simulink model "discrete_1ph_CL_VI"  (R2024a)
settings: Solver=VariableStepAuto  StartTime=0.0  StopTime=10.0  RelTol=1e-3
undefined symbols (not defined in the file): DiscIntNeverNeededParam, ILmax, kaw_i, kaw_v, ki_i, ki_v, kp_i, kp_v, Tsw, VinNom, VLlim, zden_aaf, zden_plant_i, znum_aaf, znum_plant_i
libraries: simulink x1
settings Model: Creator=marzu  LastModifiedBy=marzu

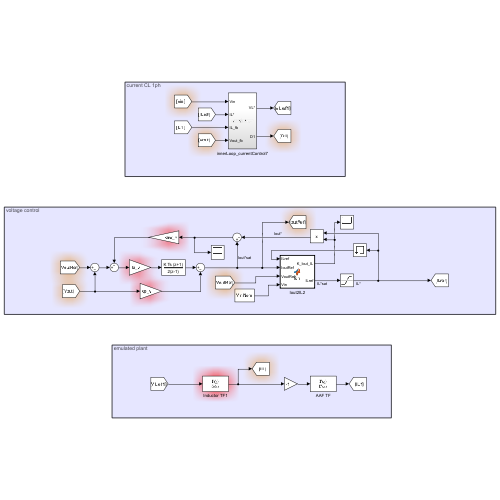
[thumbnail: Simulink's stored preview of the top-level diagram]
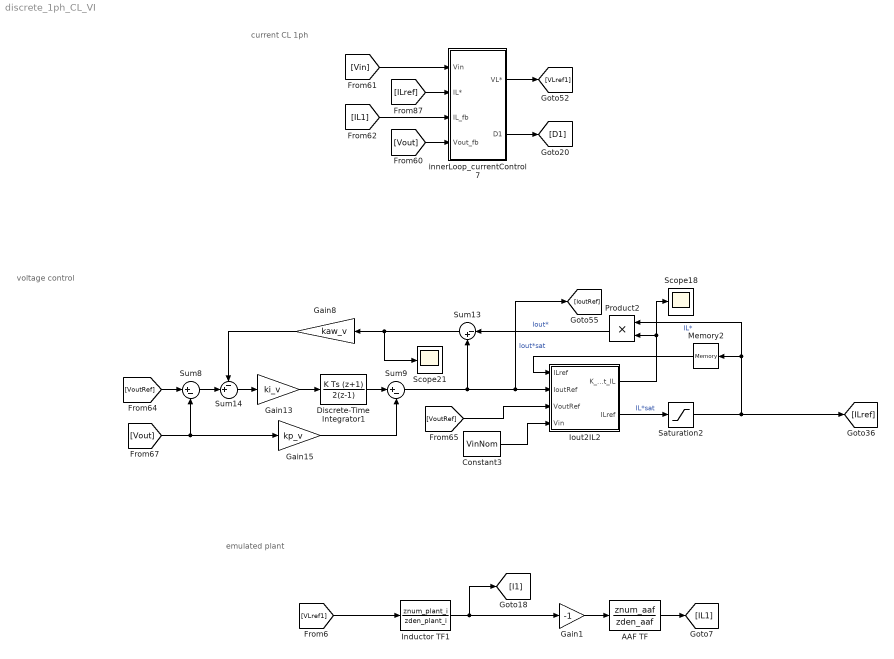
== system discrete_1ph_CL_VI ==
  note: voltage control
  note: emulated plant
  note: current CL 1ph
  AAF TF : DiscreteTransferFcn  Numerator=znum_aaf  Denominator=zden_aaf
  Constant3 : Constant  Value=VinNom
  Discrete-Time Integrator1 : DiscreteIntegrator  IntegratorMethod=Integration: Trapezoidal  SampleTime=Tsw  ICPrevOutput=DiscIntNeverNeededParam  ICPrevScaledInput=DiscIntNeverNeededParam
  Gain1 : Gain  Gain=-1
  Gain13 : Gain  Gain=ki_v
  Gain15 : Gain  Gain=kp_v
  Gain8 : Gain  Gain=kaw_v
  Inductor TF1 : DiscreteTransferFcn  Numerator=znum_plant_i  Denominator=zden_plant_i
  Iout2IL2 : MATLAB Function  TreatAsAtomicUnit=on
  Memory2 : Memory
  Product2 : Product
  Saturation2 : Saturate  UpperLimit=ILmax  LowerLimit=-ILmax
  Scope18 : Scope
  Scope21 : Scope
  Sum13 : Sum  Inputs=|-+
  Sum14 : Sum  Inputs=-+|
  Sum8 : Sum  Inputs=|+-
  Sum9 : Sum  Inputs=|+-
  innerLoop_currentControl7 : Subsystem
  wires:
  Gain1/1 -> AAF TF/1
  [VLref1] -> Inductor TF1/1
  Inductor TF1/1 -> [I1], Gain1/1
  AAF TF/1 -> [IL1]
  [Vout] -> innerLoop_currentControl7/4(Vout_fb)
  [IL1] -> innerLoop_currentControl7/3(IL_fb)
  [ILref] -> innerLoop_currentControl7/2(IL*)
  [Vin] -> innerLoop_currentControl7/1(Vin)
  innerLoop_currentControl7/2(D1) -> [D1]
  innerLoop_currentControl7/1(VL*) -> [VLref1]
  Gain13/1 -> Discrete-Time Integrator1/1
  [VoutRef] -> Sum8/1
  [Vout] -> Gain15/1, Sum8/2
  Iout2IL2/1(K_Iout_IL) -> Product2/2, Scope18/1
  Sum9/1 -> Sum13/2, Iout2IL2/2(IoutRef), [IoutRef]  "Iout*sat"
  [VoutRef] -> Iout2IL2/3(VoutRef)
  Sum14/1 -> Gain13/1
  Memory2/1 -> Iout2IL2/1("ILref ")
  Sum8/1 -> Sum14/2
  Gain15/1 -> Sum9/2
  Gain8/1 -> Sum14/1
  Constant3/1 -> Iout2IL2/4(Vin)
  Discrete-Time Integrator1/1 -> Sum9/1
  Product2/1 -> Sum13/1  "Iout*"
  Sum13/1 -> Scope21/1, Gain8/1
  Iout2IL2/2(ILref) -> Saturation2/1  "IL*sat"
  Saturation2/1 -> [ILref], Product2/1, Memory2/1  "IL*"

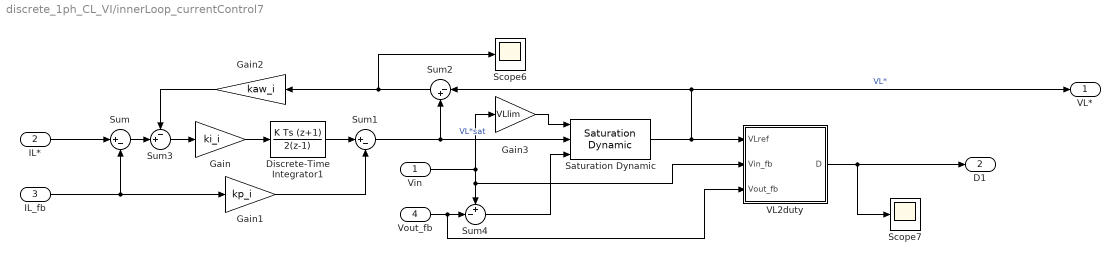
== system discrete_1ph_CL_VI/innerLoop_currentControl7 ==
  Vin : Inport
  IL* : Inport  Port=2
  IL_fb : Inport  Port=3
  Vout_fb : Inport  Port=4
  Discrete-Time Integrator1 : DiscreteIntegrator  IntegratorMethod=Integration: Trapezoidal  SampleTime=Tsw  ICPrevOutput=DiscIntNeverNeededParam  ICPrevScaledInput=DiscIntNeverNeededParam
  Gain : Gain  Gain=ki_i
  Gain1 : Gain  Gain=kp_i
  Gain2 : Gain  Gain=kaw_i
  Gain3 : Gain  Gain=VLlim
  Saturation Dynamic : simulink/Discontinuities/Saturation Dynamic  OutMin=[]  OutMax=[]  OutDataTypeStr=Inherit: Same as second input  OutDataType=fixdt(1, 16)  OutScaling=2^-10  DoSatur=off
  Scope6 : Scope
  Scope7 : Scope
  Sum : Sum  Inputs=|+-
  Sum1 : Sum  Inputs=|+-
  Sum2 : Sum  Inputs=|-+
  Sum3 : Sum  Inputs=-+|
  Sum4 : Sum  Inputs=+-|
  VL2duty : MATLAB Function  TreatAsAtomicUnit=on
  VL* : Outport
  D1 : Outport  Port=2
  wires:
  VL2duty/1(D) -> D1/1, Scope7/1
  Sum/1 -> Sum3/2
  Gain3/1 -> Saturation Dynamic/1
  Gain1/1 -> Sum1/2
  Sum3/1 -> Gain/1
  Gain/1 -> Discrete-Time Integrator1/1
  Gain2/1 -> Sum3/1
  Vin/1 -> VL2duty/2(Vin_fb), Sum4/1, Gain3/1
  Sum1/1 -> Saturation Dynamic/2, Sum2/2  "VL*sat"
  Sum4/1 -> Saturation Dynamic/3
  Sum2/1 -> Gain2/1, Scope6/1
  Saturation Dynamic/1 -> VL2duty/1(VLref), VL*/1, Sum2/1  "VL*"
  IL_fb/1 -> Sum/2, Gain1/1
  Vout_fb/1 -> VL2duty/3(Vout_fb), Sum4/2
  Discrete-Time Integrator1/1 -> Sum1/1
  IL*/1 -> Sum/1

== matlab function discrete_1ph_CL_VI/Iout2IL2 ==
  data: K_Iout_IL output; ILref input; IoutRef input; VoutRef input; Vin input; ILref output; RserL parameter
function [K_Iout_IL,ILref] = fcn(ILref,IoutRef,VoutRef,Vin,RserL)

if VoutRef < Vin
    VoutRef = Vin;
end
K_Iout_IL = (Vin - RserL*ILref) / VoutRef;
ILref = IoutRef / K_Iout_IL;

== matlab function discrete_1ph_CL_VI/innerLoop_currentControl7/VL2duty ==
  data: VLref input; D output; Vin_fb input; Vout_fb input
function D = fcn(VLref,Vin_fb,Vout_fb)

D = min([1 max([0 1 + (VLref - Vin_fb)/Vout_fb])]);
